simulink model "Modulador_de_torque_final"  (R2021a)
settings: Solver=VariableStepAuto  StartTime=0.0  StopTime=10.0  RelTol=1e-3
undefined symbols (not defined in the file): beq, g, l_cm, l_l, lambda_m, Ld, Lq, m, m_l, Pp, r, R0, Rd, Rq, Rs
settings Model: Creator=fhlla  LastModifiedBy=fhlla

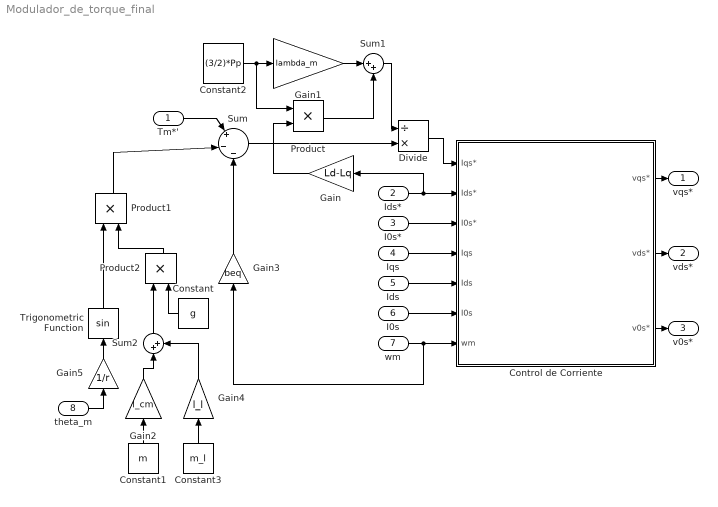
== system Modulador_de_torque_final ==
  Tm*' : Inport
  Ids* : Inport  Port=2
  I0s* : Inport  Port=3
  Iqs : Inport  Port=4
  Ids : Inport  Port=5
  I0s : Inport  Port=6
  wm : Inport  Port=7
  theta_m : Inport  Port=8
  Constant : Constant  Value=g
  Constant1 : Constant  Value=m
  Constant2 : Constant  Value=(3/2)*Pp
  Constant3 : Constant  Value=m_l
  Control de Corriente : Subsystem
  Divide : Product  Inputs=/*
  Gain : Gain  Gain=Ld-Lq
  Gain1 : Gain  Gain=lambda_m
  Gain2 : Gain  Gain=l_cm
  Gain3 : Gain  Gain=beq
  Gain4 : Gain  Gain=l_l
  Gain5 : Gain  Gain=1/r
  Product : Product
  Product1 : Product
  Product2 : Product
  Sum : Sum  Inputs=|+|-|-
  Sum1 : Sum  Inputs=|++
  Sum2 : Sum  Inputs=|++
  Trigonometric Function : Trigonometry
  vqs* : Outport
  vds* : Outport  Port=2
  v0s* : Outport  Port=3
  wires:
  Gain3/1 -> Sum/3
  Sum/1 -> Divide/2
  Divide/1 -> Control de Corriente/1(Iqs*)
  Control de Corriente/3(v0s*) -> v0s*/1
  Constant/1 -> Product2/2
  Trigonometric Function/1 -> Product1/1
  Gain2/1 -> Sum2/1
  Sum2/1 -> Product2/1
  Product2/1 -> Product1/2
  Product1/1 -> Sum/2
  Gain5/1 -> Trigonometric Function/1
  Tm*'/1 -> Sum/1
  Gain1/1 -> Sum1/1
  theta_m/1 -> Gain5/1
  Gain/1 -> Product/2
  Iqs/1 -> Control de Corriente/4(Iqs)
  Constant2/1 -> Gain1/1, Product/1
  Control de Corriente/1(vqs*) -> vqs*/1
  Control de Corriente/2(vds*) -> vds*/1
  I0s/1 -> Control de Corriente/6(I0s)
  I0s*/1 -> Control de Corriente/3(I0s*)
  Gain4/1 -> Sum2/2
  Ids*/1 -> Gain/1, Control de Corriente/2(Ids*)
  Constant1/1 -> Gain2/1
  Constant3/1 -> Gain4/1
  Product/1 -> Sum1/2
  Sum1/1 -> Divide/1
  wm/1 -> Gain3/1, Control de Corriente/7(wm)
  Ids/1 -> Control de Corriente/5(Ids)

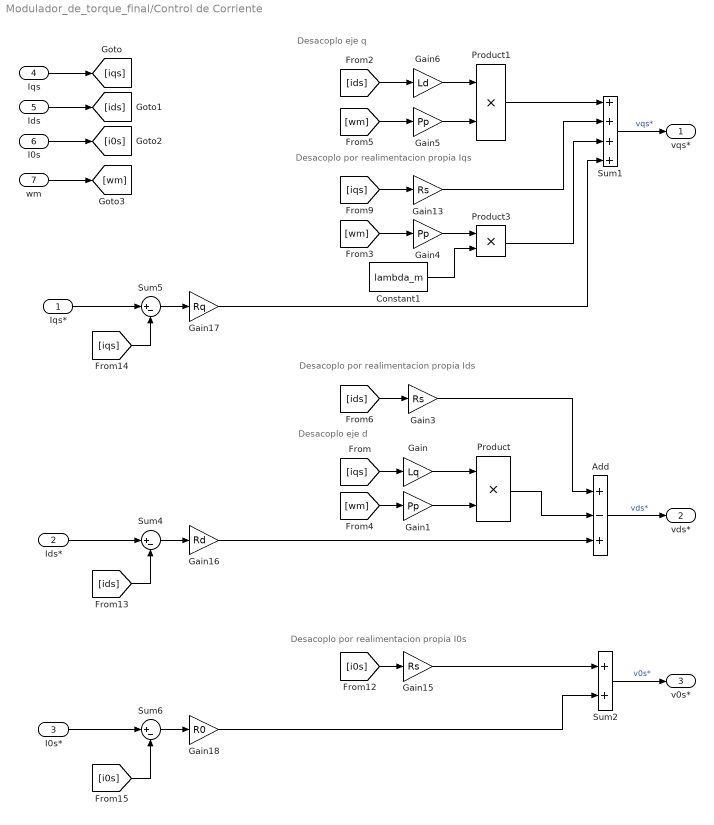
== system Modulador_de_torque_final/Control de Corriente ==
  note: Desacoplo por realimentacion propia I0s
  note: Desacoplo por realimentacion propia Iqs
  note: Desacoplo por realimentacion propia Ids
  note: Desacoplo eje d
  note: Desacoplo eje q
  Iqs* : Inport
  Ids* : Inport  Port=2
  I0s* : Inport  Port=3
  Iqs : Inport  Port=4
  Ids : Inport  Port=5
  I0s : Inport  Port=6
  wm : Inport  Port=7
  Add : Sum  Inputs=+-+
  Constant1 : Constant  Value=lambda_m
  Gain : Gain  Gain=Lq
  Gain1 : Gain  Gain=Pp
  Gain13 : Gain  Gain=Rs
  Gain15 : Gain  Gain=Rs
  Gain16 : Gain  Gain=Rd
  Gain17 : Gain  Gain=Rq
  Gain18 : Gain  Gain=R0
  Gain3 : Gain  Gain=Rs
  Gain4 : Gain  Gain=Pp
  Gain5 : Gain  Gain=Pp
  Gain6 : Gain  Gain=Ld
  Product : Product
  Product1 : Product
  Product3 : Product
  Sum1 : Sum  Inputs=++++
  Sum2 : Sum
  Sum4 : Sum  Inputs=|+-
  Sum5 : Sum  Inputs=|+-
  Sum6 : Sum  Inputs=|+-
  vqs* : Outport
  vds* : Outport  Port=2
  v0s* : Outport  Port=3
  wires:
  [i0s] -> Sum6/2
  Sum2/1 -> v0s*/1  "v0s*"
  Iqs*/1 -> Sum5/1
  I0s*/1 -> Sum6/1
  [iqs] -> Gain13/1
  [ids] -> Sum4/2
  [i0s] -> Gain15/1
  Sum5/1 -> Gain17/1
  [iqs] -> Sum5/2
  [ids] -> Gain3/1
  Gain13/1 -> Sum1/2
  Sum6/1 -> Gain18/1
  Ids*/1 -> Sum4/1
  Gain15/1 -> Sum2/1
  Gain18/1 -> Sum2/2
  Gain17/1 -> Sum1/4
  Product1/1 -> Sum1/1
  Product/1 -> Add/2
  Gain5/1 -> Product1/2
  Gain/1 -> Product/1
  Gain4/1 -> Product3/1
  Sum4/1 -> Gain16/1
  Constant1/1 -> Product3/2
  Product3/1 -> Sum1/3
  Add/1 -> vds*/1  "vds*"
  Sum1/1 -> vqs*/1  "vqs*"
  Iqs/1 -> [iqs]
  Ids/1 -> [ids]
  I0s/1 -> [i0s]
  [iqs] -> Gain/1
  Gain1/1 -> Product/2
  [wm] -> Gain1/1
  wm/1 -> [wm]
  [wm] -> Gain4/1
  [wm] -> Gain5/1
  [ids] -> Gain6/1
  Gain6/1 -> Product1/1
  Gain16/1 -> Add/3
  Gain3/1 -> Add/1
